simulink model "sine_gen"  (R2024b)
settings: Solver=FixedStepDiscrete  StartTime=0.0  StopTime=10/50  RelTol=1e-3
InitFcn:
  | f_sim=1/2e6;
  | fsw = 65;             % kHz
  | tsw = 1/(fsw*1e3);    % sec
  | t_ss = tsw/30;        % sec
libraries: dspsrcs4 x3
settings Model: DataTypeOverride=Off  Creator=angro  LastModifiedBy=Angel
settings OptimizationCC: BlockReduction=off  ConditionallyExecuteInputs=off  DefaultParameterBehavior=Inlined  InheritOutputTypeSmallerThanSingle=on
settings DebuggingCC: ArtificialAlgebraicLoopMsg=error  SingleTaskRateTransMsg=error
settings HardwareCC: ProdBitPerPointer=32  ProdBitPerSizeT=32  ProdBitPerPtrDiffT=32  ProdLargestAtomicFloat=None  ProdIntDivRoundTo=Undefined  ProdEndianess=Unspecified  ProdWordSize=32  ProdHWDeviceType=ASIC/FPGA->ASIC/FPGA  TargetBitPerPointer=64  TargetBitPerSizeT=64  TargetBitPerPtrDiffT=64  TargetLongLongMode=on  TargetIntDivRoundTo=Zero  TargetEndianess=LittleEndian  TargetWordSize=64  TargetHWDeviceType=Custom Processor->MATLAB Host Computer  ProdEqTarget=off

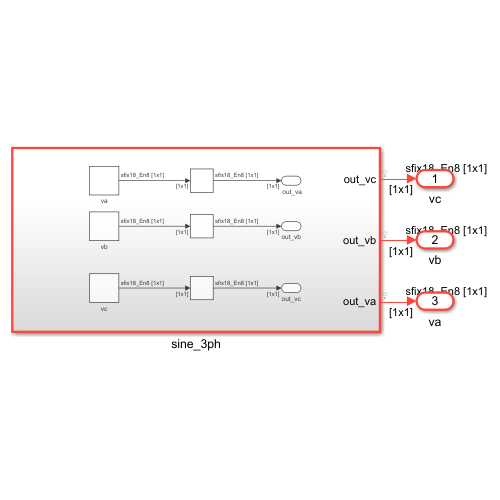
[thumbnail: Simulink's stored preview of the top-level diagram]
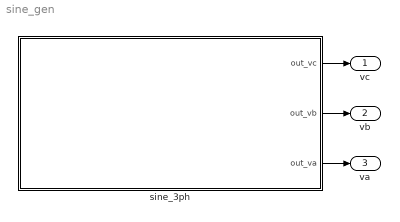
== system sine_gen ==
  sine_3ph : Subsystem
  vc : Outport
  vb : Outport  Port=2
  va : Outport  Port=3
  wires:
  sine_3ph/1(out_vc) -> vc/1
  sine_3ph/2(out_vb) -> vb/1
  sine_3ph/3(" out_va") -> va/1

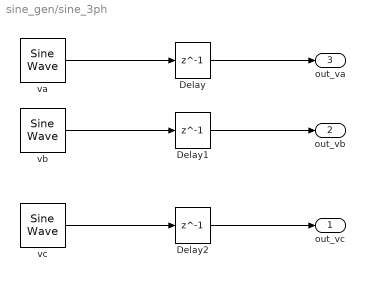
== system sine_gen/sine_3ph ==
  Delay : Delay  DelayLength=1  InputProcessing=Columns as channels (frame based)
  Delay1 : Delay  DelayLength=1  InputProcessing=Columns as channels (frame based)
  Delay2 : Delay  DelayLength=1  InputProcessing=Columns as channels (frame based)
  va : dspsrcs4/Sine Wave  Amplitude=325  Frequency=50  Phase=0  SampleMode=Discrete  OutComplex=Real  CompMethod=Table lookup  TableSize=Speed  SampleTime=1/4.7e3  SamplesPerFrame=1  ResetState=Restart at time zero  OutputFrames=off  dataType=Fixed-point  wordLen=18  udDataType=sfix(16)  fracBitsMode=User-defined  numFracBits=8  OutDataTypeStr=fixdt(1,18,8)  LastOutDataTypeStr=fixdt(1,18,8)
  vb : dspsrcs4/Sine Wave  Amplitude=325  Frequency=50  Phase=-2*pi/3  SampleMode=Discrete  OutComplex=Real  CompMethod=Table lookup  TableSize=Speed  SampleTime=1/4.7e3  SamplesPerFrame=1  ResetState=Restart at time zero  OutputFrames=off  dataType=Fixed-point  wordLen=18  udDataType=sfix(16)  fracBitsMode=User-defined  numFracBits=8  OutDataTypeStr=fixdt(1,18,8)  LastOutDataTypeStr=fixdt(1,18,8)
  vc : dspsrcs4/Sine Wave  Amplitude=325  Frequency=50  Phase=2*pi/3  SampleMode=Discrete  OutComplex=Real  CompMethod=Table lookup  TableSize=Speed  SampleTime=1/4.7e3  SamplesPerFrame=1  ResetState=Restart at time zero  OutputFrames=off  dataType=Fixed-point  wordLen=18  udDataType=sfix(16)  fracBitsMode=User-defined  numFracBits=8  OutDataTypeStr=fixdt(1,18,8)  LastOutDataTypeStr=fixdt(1,18,8)
  out_vc : Outport
  out_vb : Outport  Port=2
  " out_va" : Outport  Port=3
  wires:
  va/1 -> Delay/1
  vb/1 -> Delay1/1
  vc/1 -> Delay2/1
  Delay/1 -> " out_va"/1
  Delay1/1 -> out_vb/1
  Delay2/1 -> out_vc/1
